simulink model "simulink_FCS_SDA"  (R2023a)
settings: Solver=VariableStepAuto  StartTime=0.0  StopTime=3*(1/freqHzSin)  FixedStep=Ts  RelTol=1e-3
InitFcn:
  | % try
  | %     Excel = actxGetRunningServer('Excel.Application');
  | %     Excel.ActiveWorkbook.Save;
  | %     Excel.ActiveWorkbook.Close(false);
  | % catch ExcelFechado
  | % end
StopFcn:
  | % t = table(out.seq, out.t_sim, 'VariableNames', ["Sequência de Vetores","Tempo de Simulação"]);
  | % writetable(t,'C:\Users\jpbru\OneDrive\Documentos\UFSC\COBEP 2023\sequencia_states.xlsx','Sheet','sim_CF_gw')
  | % winopen('C:\Users\jpbru\OneDrive\Documentos\UFSC\COBEP 2023\sequencia_states.xlsx')
  | %
  | % nome_arq = sprintf("gdq_caso-1_7.csv");
  | % writematrix([out.y_d out.y_q out.y_a out.y_b out.y_c out.ref_a out.ref_b out.ref_c],"C:\Users\jpbru\OneDrive\Documentos\MATLAB\CPBM\TrabFinal\Etapa 9 - Setembro2023 -\graficos\"+nome_arq)
  | 
  | sprintf("THD = %.3f", out.thd)
  | sprintf("MSE = %.3f", out.mse)
  | sprintf("Csw = %.0f", out.csw)
  | sprintf("Tempo de Computo = %.3fms", out.tavg*1000)
undefined symbols (not defined in the file or in its folder): A, B, Csim, dimA, dimB, DiscIntNeverNeededParam, freqHzSin, Lfilter, Lsim, N, N1, N2, Nu, Rsim, states, Ts, Vdc, Vdc_sim, Vnoise, Vref_pico, x_enb
libraries: dspstat3 x9, spsSeriesRLCBranchLib x9, spsVoltageMeasurementLib x7, spsIdealSwitchLib x6, spsTHDLib x4, simulink x2, spsabctoAlphaBetaZeroLib x2, spsAlphaBetaZerotoabcLib x1, spsControlledVoltageSourceLib x1, spspowerguiLib x1
settings Model: Creator=jpbru  LastModifiedBy=jpbru
settings SolverCC: AlgebraicLoopSolver=TrustRegion
settings DebuggingCC: UnconnectedInputMsg=warning  UnconnectedOutputMsg=warning  UnconnectedLineMsg=warning
settings ModelReferenceCC: EnableRefExpFcnMdlSchedulingChecks=on

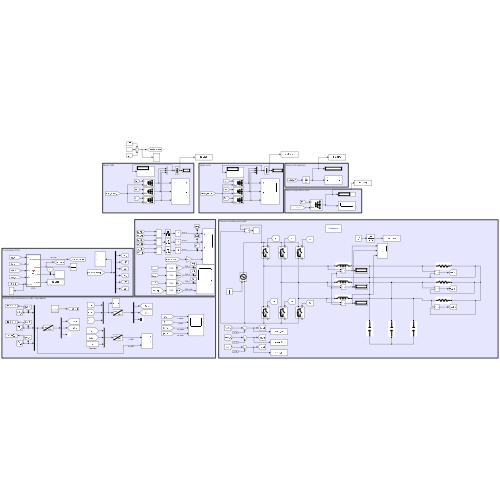
[thumbnail: Simulink's stored preview of the top-level diagram]
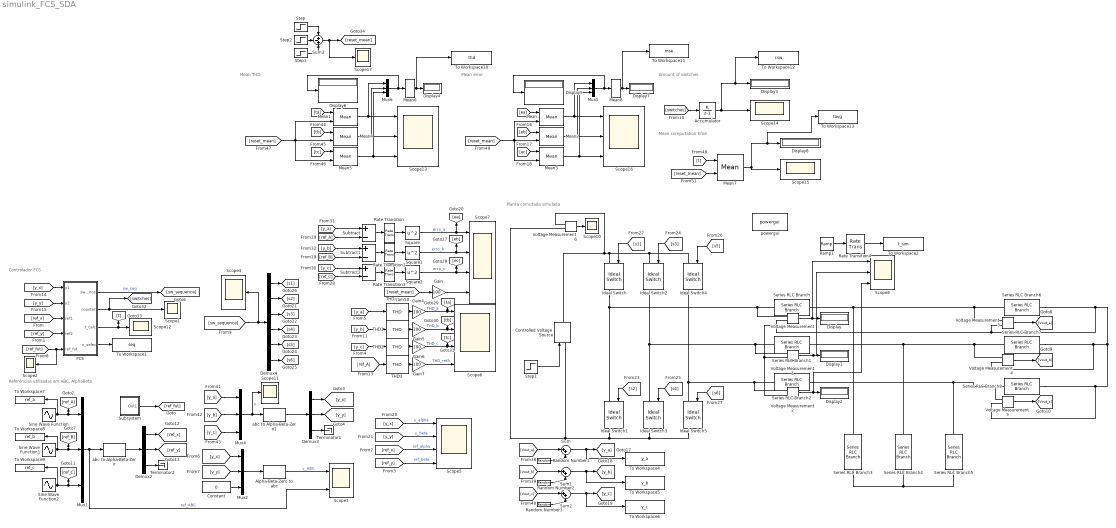
== system simulink_FCS_SDA ==
  note: Planta comutada simulada
  note: Referências utilizadas em ABC, AlphaBeta
  note: Controlador FCS
  note: Mean computation time
  note: Mean error
  note: Amount of switches
  note: Mean THD
  Accumulator : DiscreteIntegrator  IntegratorMethod=Accumulation: Forward Euler  SampleTime=-1  ICPrevOutput=DiscIntNeverNeededParam  ICPrevScaledInput=DiscIntNeverNeededParam
  Alpha-Beta-Zero to abc : spsAlphaBetaZerotoabcLib/Alpha-Beta-Zero to abc
      settings: LibrarySourceBlock=|
      | sps_lib/Control/Alpha-Beta-Zero
      | to abc
  Constant : Constant  Value=0  VectorParams1D=off  SampleTime=-1
  Controlled Voltage Source : spsControlledVoltageSourceLib/Controlled Voltage Source  Initialize=on  Source_Type=DC  Amplitude=Vdc_sim  Phase=0  Frequency=0  Measurements=None
  Demux2 : Demux  Outputs=3
  Demux3 : Demux  Outputs=3
  Demux4 : Demux  Outputs=6
  Display{,1..8} (9 alike) : Display
      Display8 settings: Format=short_e
  FCS : MATLAB Function  TreatAsAtomicUnit=on  SystemSampleTime=Ts
  Gain{,4..7} (5 alike) : Gain  Gain=100
  Ideal Switch{,1..5} (6 alike) : spsIdealSwitchLib/Ideal Switch  Ron=0.001  Lon=0  IC=0  Rs=1e5  Cs=inf  Measurements=on
  Mean{,1..5,7} (7 alike) : dspstat3/Mean  run=on  reset_popup=Rising edge  directionMode=Each column  dimension=1  roiEnable=off  roiType=Rectangles  roiPortion=Entire ROI  roiOutput=Individual statistics for each ROI  roiFlag=off  roundingMode=Floor  overflowMode=off  outputDataTypeStr=Inherit: Same as accumulator  outputMin=[]  outputMax=[]  outputLastDataTypeStr=Inherit: Same as accumulator
  Mean6 : dspstat3/Mean  run=off  reset_popup=Rising edge  directionMode=Entire input  dimension=1  roiEnable=off  roiType=Rectangles  roiPortion=Entire ROI  roiOutput=Individual statistics for each ROI  roiFlag=off  roundingMode=Floor  overflowMode=off  outputDataTypeStr=Inherit: Same as accumulator  outputMin=[]  outputMax=[]  outputLastDataTypeStr=Inherit: Same as accumulator
  Mean8 : dspstat3/Mean  run=off  reset_popup=Rising edge  directionMode=Entire input  dimension=1  roiEnable=off  roiType=Rectangles  roiPortion=Entire ROI  roiOutput=Individual statistics for each ROI  roiFlag=off  roundingMode=Floor  overflowMode=off  outputDataTypeStr=Inherit: Same as accumulator  outputMin=[]  outputMax=[]  outputLastDataTypeStr=Inherit: Same as accumulator
  Mux{1..2,4..6} (5 alike) : Mux  Inputs=3
  Ramp1 : simulink/Sources/Ramp  slope=1  start=0  InitialOutput=0
  Random Number1 : RandomNumber  Variance=Vnoise  SampleTime=Ts
  Random Number2 : RandomNumber  Variance=Vnoise  SampleTime=Ts
  Random Number3 : RandomNumber  Variance=Vnoise  SampleTime=Ts
  Rate Transition{,2..4} (4 alike) : RateTransition  OutPortSampleTime=Ts
  Scope{1..2,4,10..12,14..15,17} (9 alike) : Scope
  Scope13 : Scope  NumInputPorts=3
  Scope16 : Scope  NumInputPorts=3
  Scope3 : Scope  NumInputPorts=2
  Scope5 : Scope  NumInputPorts=4
  Scope6 : Scope  NumInputPorts=4
  Scope7 : Scope  NumInputPorts=4
  Scope8 : Scope  NumInputPorts=3
  Series RLC Branch : spsSeriesRLCBranchLib/Series RLC Branch  LConnTagsString=__new0  RConnTagsString=__new0  BranchType=L  Resistance=1  Inductance=Lsim  SetiL0=off  InitialCurrent=0  Capacitance=1e-6  Setx0=off  InitialVoltage=0  Measurements=None
  Series RLC Branch1 : spsSeriesRLCBranchLib/Series RLC Branch  LConnTagsString=__new0  RConnTagsString=__new0  BranchType=L  Resistance=1  Inductance=Lsim  SetiL0=off  InitialCurrent=0  Capacitance=1e-6  Setx0=off  InitialVoltage=0  Measurements=None
  Series RLC Branch2 : spsSeriesRLCBranchLib/Series RLC Branch  LConnTagsString=__new0  RConnTagsString=__new0  BranchType=L  Resistance=1  Inductance=Lsim  SetiL0=off  InitialCurrent=0  Capacitance=1e-6  Setx0=off  InitialVoltage=0  Measurements=None
  Series RLC Branch3 : spsSeriesRLCBranchLib/Series RLC Branch  LConnTagsString=__new0  RConnTagsString=__new0  BranchType=C  Resistance=1  Inductance=1e-3  SetiL0=off  InitialCurrent=0  Capacitance=Csim  Setx0=off  InitialVoltage=0  Measurements=None
  Series RLC Branch4 : spsSeriesRLCBranchLib/Series RLC Branch  LConnTagsString=__new0  RConnTagsString=__new0  BranchType=C  Resistance=1  Inductance=1e-3  SetiL0=off  InitialCurrent=0  Capacitance=Csim  Setx0=off  InitialVoltage=0  Measurements=None
  Series RLC Branch5 : spsSeriesRLCBranchLib/Series RLC Branch  LConnTagsString=__new0  RConnTagsString=__new0  BranchType=C  Resistance=1  Inductance=1e-3  SetiL0=off  InitialCurrent=0  Capacitance=Csim  Setx0=off  InitialVoltage=0  Measurements=None
  Series RLC Branch6 : spsSeriesRLCBranchLib/Series RLC Branch  LConnTagsString=__new0  RConnTagsString=__new0  BranchType=R  Resistance=Rsim  Inductance=Lfilter  SetiL0=off  InitialCurrent=0  Capacitance=1e-6  Setx0=off  InitialVoltage=0  Measurements=None
  Series RLC Branch7 : spsSeriesRLCBranchLib/Series RLC Branch  LConnTagsString=__new0  RConnTagsString=__new0  BranchType=R  Resistance=Rsim  Inductance=Lfilter  SetiL0=off  InitialCurrent=0  Capacitance=1e-6  Setx0=off  InitialVoltage=0  Measurements=None
  Series RLC Branch8 : spsSeriesRLCBranchLib/Series RLC Branch  LConnTagsString=__new0  RConnTagsString=__new0  BranchType=R  Resistance=Rsim  Inductance=Lfilter  SetiL0=off  InitialCurrent=0  Capacitance=1e-6  Setx0=off  InitialVoltage=0  Measurements=None
  Sine Wave Function : Sin  Amplitude=Vref_pico  Frequency=2*pi*50  SampleTime=Ts
  Sine Wave Function1 : Sin  Amplitude=Vref_pico  Frequency=2*pi*50  Phase=-2*pi/3  SampleTime=Ts
  Sine Wave Function2 : Sin  Amplitude=Vref_pico  Frequency=2*pi*50  Phase=2*pi/3  SampleTime=Ts
  Square : Math  Operator=square
  Square1 : Math  Operator=square
  Square2 : Math  Operator=square
  Step : Step  Time=(1/freqHzSin)  SampleTime=Ts
  Step1 : Step  Time=0.5  Before=Vdc_sim  After=Vdc_sim  SampleTime=Ts
  Step2 : Step  Time=(1/freqHzSin)+Ts  SampleTime=Ts
  Step3 : Step  Time=(1/freqHzSin)*2  SampleTime=Ts
  Subsystem : Subsystem
  Subtract : Sum  Inputs=+-
  Subtract1 : Sum  Inputs=+-
  Subtract2 : Sum  Inputs=+-
  Sum : Sum  Inputs=|++
  Sum1 : Sum  Inputs=|++
  Sum2 : Sum  Inputs=|++
  Sum3 : Sum  Inputs=+-+
  THD{,1..3} (4 alike) : spsTHDLib/THD  Freq=50  Ts=Ts
  Terminator1 : Terminator
  Terminator2 : Terminator
  To Workspace1 : ToWorkspace  VariableName=seq  SampleTime=Ts
      settings: Save2DSignal=2-D array (concatenate along first dimension)
  To Workspace10 : ToWorkspace  VariableName=thd  SampleTime=-1
      settings: MaxDataPoints=1
  To Workspace11 : ToWorkspace  VariableName=mse  SampleTime=-1
      settings: MaxDataPoints=1
  To Workspace12 : ToWorkspace  VariableName=csw  SampleTime=-1
      settings: MaxDataPoints=1
  To Workspace13 : ToWorkspace  VariableName=tavg  SampleTime=-1
      settings: MaxDataPoints=1
  To Workspace2 : ToWorkspace  VariableName=t_sim  SampleTime=Ts
      settings: Save2DSignal=2-D array (concatenate along first dimension)
  To Workspace4 : ToWorkspace  VariableName=y_a  SampleTime=Ts
      settings: Save2DSignal=2-D array (concatenate along first dimension)
  To Workspace5 : ToWorkspace  VariableName=y_b  SampleTime=Ts
      settings: Save2DSignal=2-D array (concatenate along first dimension)
  To Workspace6 : ToWorkspace  VariableName=y_c  SampleTime=Ts
      settings: Save2DSignal=2-D array (concatenate along first dimension)
  To Workspace7 : ToWorkspace  VariableName=ref_a  SampleTime=Ts
      settings: Save2DSignal=2-D array (concatenate along first dimension)
  To Workspace8 : ToWorkspace  VariableName=ref_b  SampleTime=Ts
      settings: Save2DSignal=2-D array (concatenate along first dimension)
  To Workspace9 : ToWorkspace  VariableName=ref_c  SampleTime=Ts
      settings: Save2DSignal=2-D array (concatenate along first dimension)
  Voltage Measurement{,1..6} (7 alike) : spsVoltageMeasurementLib/Voltage Measurement  PhasorSimulation=off  OutputType=Complex  PSBequivalent=0
  abc to Alpha-Beta-Zero : spsabctoAlphaBetaZeroLib/abc to Alpha-Beta-Zero
  abc to Alpha-Beta-Zero1 : spsabctoAlphaBetaZeroLib/abc to Alpha-Beta-Zero
  powergui : spspowerguiLib/powergui  Priority=1  SimulationMode=Continuous  SampleTime=Ts  frequency=60  Iterations=50  frequencyindice=0  Pbase=100e6  ErrMax=1e-4  UnitsV=kV  UnitsW=MW  buscounter=0  FunctionMessages=off  echomessages=off  EnableUseOfTLC=off  CurrentSourceSwitches=off  DisableSnubberDevices=off  DisableRonSwitches=off  DisableVfSwitches=off  DisplayEquations=off  AutomaticDiscreteSolvers=off  SolverType=Tustin/Backward Euler (TBE)  Interpol=off  ExternalGateDelay=off  methode=off  Ts=100  x0status=blocks  SPID=on  SwTol=0  HookPort=off  NonlinearTolerance=1e-4  nMaxIteration=100  ContinueOnMaxIteration=off  RestoreLinks=warning  ResistiveCurrentMeasurement=off  Frange=[0:2:500]  Ylog=off  Xlog=on  ShowGrid=off  save=off  variable=ZData  structure=0  ZoomFFT=off  StartTime=0.0  cycles=1  DisplayStyle=1  fundamental=60  FreqAxis=off  MaxFrequency=1000  frequencyindicesteady=1  RmsSteady=1  display=off
  wires:
  [ref_y] -> Scope5/4  "ref_beta"
  Sine Wave Function/1 -> Mux1/1, [ref_A], To Workspace7/1
  Sine Wave Function1/1 -> [ref_B], Mux1/2, To Workspace8/1
  Sine Wave Function2/1 -> [ref_C], Mux1/3, To Workspace9/1
  Mux1/1 -> Scope3/2, abc to Alpha-Beta-Zero/1  "ref_ABC"
  [y_x] -> Mux2/1
  [y_y] -> Mux2/2
  Constant/1 -> Mux2/3
  Alpha-Beta-Zero to abc/1 -> Scope3/1  "y_ABC"
  Voltage Measurement2/1 -> Scope8/3, Display2/1
  Voltage Measurement/1 -> Scope8/1, Display/1
  Voltage Measurement3/1 -> [Vout_a]
  Voltage Measurement4/1 -> [Vout_b]
  Voltage Measurement1/1 -> Scope8/2, Display1/1
  Voltage Measurement5/1 -> [Vout_c]
  [y_b] -> Mux4/2
  [y_a] -> Mux4/1
  [y_c] -> Mux4/3
  abc to Alpha-Beta-Zero1/1 -> Demux3/1
  Demux3/1 -> [y_x]
  Demux3/2 -> [y_y]
  [y_x] -> Scope5/1  "y_alpha"
  [y_y] -> Scope5/2  "y_beta"
  Demux3/3 -> Terminator1/1
  [s6] -> Ideal Switch5/1
  [s1] -> Ideal Switch/1
  [s2] -> Ideal Switch1/1
  [s3] -> Ideal Switch2/1
  [s5] -> Ideal Switch4/1
  [s4] -> Ideal Switch3/1
  Demux4/3 -> [s3]
  Demux4/1 -> [s1]
  Demux4/2 -> [s2]
  Demux4/5 -> [s5]
  Demux4/6 -> [s6]
  Demux4/4 -> [s4]
  [sw_sequence] -> Scope4/1, Demux4/1
  FCS/1(sw_sequence) -> [sw_sequence]  "sw_seq"
  [y_x] -> FCS/1(y1)
  [y_y] -> FCS/2(y2)
  [ref_x] -> FCS/3(ref1)
  [ref_y] -> FCS/4(ref2)
  FCS/2(counter) -> [switches], Scope1/1
  [ref_x] -> Scope5/3  "ref_alpha"
  Demux2/2 -> [ref_y]
  Demux2/1 -> [ref_x]
  Demux2/3 -> Terminator2/1
  abc to Alpha-Beta-Zero/1 -> Demux2/1
  Mux4/1 -> Scope11/1, abc to Alpha-Beta-Zero1/1  "y"
  Mux2/1 -> Alpha-Beta-Zero to abc/1
  Subsystem/1(Out1) -> [ref_fut]
  [ref_fut] -> Scope2/1, FCS/5(ref_fut)
  Voltage Measurement6/1 -> Scope10/1
  [Vout_b] -> Sum1/1
  Sum2/1 -> To Workspace6/1, [y_c]
  Sum/1 -> To Workspace4/1, [y_a]
  Random Number1/1 -> Sum/2
  Random Number2/1 -> Sum1/2
  Random Number3/1 -> Sum2/2
  Sum1/1 -> To Workspace5/1, [y_b]
  [Vout_a] -> Sum/1
  [Vout_c] -> Sum2/1
  FCS/3(t_calc) -> [t], Scope12/1
  [t] -> Mean7/1
  Mean7/1 -> To Workspace13/1, Display8/1, Scope15/1
  [ea] -> Mean/1
  [ec] -> Mean3/1
  Mux5/1 -> Mean8/1, Display5/1
  Mean/1 -> Mux5/1, Scope16/1
  Mean3/1 -> Mux5/3, Scope16/3
  Mean2/1 -> Mux5/2, Scope16/2
  [eb] -> Mean2/1
  THD/1 -> Gain4/1
  Square1/1 -> [eb], Scope7/2  "erro_b"
  [y_b] -> THD1/1
  [ref_B] -> Subtract1/2
  Gain5/1 -> [tb], Scope6/2  "THD_b"
  [y_c] -> Subtract2/1
  [y_b] -> Subtract1/1
  [ref_C] -> Subtract2/2
  [y_a] -> Subtract/1
  [ref_A] -> THD3/1
  THD1/1 -> Gain5/1
  Gain7/1 -> Scope6/4  "THD_refA"
  Subtract1/1 -> Rate Transition2/1
  THD2/1 -> Gain6/1
  Square2/1 -> [ec], Scope7/3  "erro_c"
  [ref_A] -> Subtract/2
  THD3/1 -> Gain7/1
  Gain6/1 -> [tc], Scope6/3  "THD_c"
  Subtract2/1 -> Rate Transition3/1
  [y_a] -> THD/1
  Subtract/1 -> Rate Transition/1
  Square/1 -> [ea], Scope7/1  "erro_a"
  [y_c] -> THD2/1
  Gain4/1 -> [ta], Scope6/1  "THD_a"
  Accumulator/1 -> To Workspace12/1, Display3/1, Scope14/1
  [switches] -> Accumulator/1
  [tc] -> Mean5/1
  [ta] -> Mean1/1
  Mean5/1 -> Mux6/3, Scope13/3
  Mean4/1 -> Mux6/2, Scope13/2
  [tb] -> Mean4/1
  Mux6/1 -> Display6/1, Mean6/1
  Mean1/1 -> Mux6/1, Scope13/1
  Rate Transition/1 -> Square/1
  Rate Transition2/1 -> Square1/1
  Rate Transition3/1 -> Square2/1
  [reset_mean] -> Mean1/2, Mean5/2, Mean4/2
  [reset_mean] -> Mean3/2, Mean2/2, Mean/2
  [reset_mean] -> Gain/1
  Gain/1 -> Scope7/4
  [reset_mean] -> Mean7/2
  Mean6/1 -> To Workspace10/1, Display4/1
  Mean8/1 -> To Workspace11/1, Display7/1
  Step1/1 -> Controlled Voltage Source/1
  FCS/4(x_selec) -> To Workspace1/1
  Ramp1/1 -> Rate Transition4/1
  Rate Transition4/1 -> To Workspace2/1
  Step/1 -> Sum3/1
  Step3/1 -> Sum3/3
  Step2/1 -> Sum3/2
  Sum3/1 -> Scope17/1, [reset_mean]
  connections:
  Ideal Switch3/LConn1 -- Ideal Switch2/RConn1 -- Voltage Measurement1/LConn1 -- Series RLC Branch1/LConn1
  Ideal Switch/RConn1 -- Ideal Switch1/LConn1 -- Voltage Measurement/LConn1 -- Series RLC Branch/LConn1
  Series RLC Branch6/RConn1 -- Voltage Measurement2/LConn2 -- Voltage Measurement1/LConn2 -- Voltage Measurement/LConn2 -- Voltage Measurement3/LConn2 -- Voltage Measurement4/LConn2 -- Series RLC Branch7/RConn1 -- Voltage Measurement5/LConn2 -- Series RLC Branch8/RConn1
  Ideal Switch5/LConn1 -- Ideal Switch4/RConn1 -- Voltage Measurement2/LConn1 -- Series RLC Branch2/LConn1
  Series RLC Branch3/RConn1 -- Series RLC Branch5/RConn1 -- Series RLC Branch4/RConn1
  Series RLC Branch/RConn1 -- Series RLC Branch3/LConn1 -- Series RLC Branch6/LConn1 -- Voltage Measurement3/LConn1
  Voltage Measurement5/LConn1 -- Series RLC Branch5/LConn1 -- Series RLC Branch2/RConn1 -- Series RLC Branch8/LConn1
  Voltage Measurement4/LConn1 -- Series RLC Branch4/LConn1 -- Series RLC Branch1/RConn1 -- Series RLC Branch7/LConn1
  Ideal Switch/LConn1 -- Controlled Voltage Source/RConn1 -- Voltage Measurement6/LConn1 -- Ideal Switch4/LConn1 -- Ideal Switch2/LConn1
  Ideal Switch1/RConn1 -- Controlled Voltage Source/LConn1 -- Voltage Measurement6/LConn2 -- Ideal Switch5/RConn1 -- Ideal Switch3/RConn1

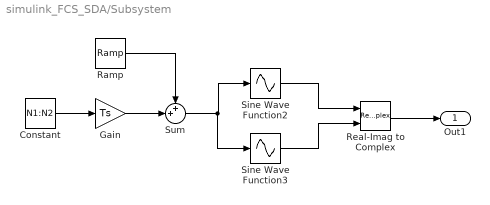
== system simulink_FCS_SDA/Subsystem ==
  Constant : Constant  Value=N1:N2
  Gain : Gain  Gain=Ts
  Ramp : simulink/Sources/Ramp  slope=1  start=0  InitialOutput=0
  Real-Imag to Complex : RealImagToComplex
  Sine Wave Function2 : Sin  TimeSource=Use external signal  Amplitude=Vref_pico  Frequency=2*pi*50  SampleTime=Ts
  Sine Wave Function3 : Sin  TimeSource=Use external signal  Amplitude=Vref_pico  Frequency=2*pi*50  Phase=-pi/2  SampleTime=Ts
  Sum : Sum  Inputs=++|
  Out1 : Outport
  wires:
  Sine Wave Function3/1 -> Real-Imag to Complex/2
  Sine Wave Function2/1 -> Real-Imag to Complex/1
  Sum/1 -> Sine Wave Function3/1, Sine Wave Function2/1
  Ramp/1 -> Sum/1
  Gain/1 -> Sum/2
  Real-Imag to Complex/1 -> Out1/1
  Constant/1 -> Gain/1

== matlab function simulink_FCS_SDA/FCS ==
  settings: updateMethod=DISCRETE  sampleTime=Ts
  data: y1 input; y2 input; ref1 input; ref2 input; ref_fut input size=N; dimA parameter; sw_sequence output; dimB parameter; states parameter; A parameter; Vdc parameter; counter output; Ts parameter; B parameter; t_calc output; N parameter; x_selec output; N1 parameter; Nu parameter; x_enb parameter
%function[variáveis que envia pra fora do bloco na simulação] = fcn(entradas(com conexões físicas) e parâmetros(que são pegos da workspace))
function [sw_sequence, counter, t_calc, x_selec] = fcn(y1, y2, ref1, ref2, ref_fut, dimA, dimB, states, A, Vdc, Ts, B, N, N1, Nu, x_enb) 
persistent t k pc pe1 pe2 pw1 pw2 y_ant u_ant a x_ant erro_intDQ u_ab %variáveis que mantém o valor entre os loops
if isempty(t) %caso t ainda não tenha valor definido
    t = 0; %o primeiro loop assume t=0
    k = 0; %variável que vai contar quantos loops são feitos para o cálculo de control
    
    %PARÂMETROS DE SINTONIZAÇÃO DO FCS-MPC
    pc = 0.35; %define o peso das comutações - quanto maior, menos comutações serão executadas durante o tempo de simulação 
    pe1 = 1; %define o peso do erro em D - quanto maior, menor deve ser o erro em D 
    pe2 = 1; %define o peso do erro em Q - quanto maior, menor deve ser o erro em Q 
    pw1 = 0; %define o peso do erro acumulado em D - quanto maior, menor deve ser o erro acumulado em D 
    pw2 = 0; %define o peso do erro acumulado em Q - quanto maior, menor deve ser o erro acumulado em Q

    a = exp(1j*(2*pi/3)); %define a variável que transforma os estados do inversor em uma variável complexa
    y_ant = complex(zeros(dimA-1,1)); %inicializa o vetor complexo com a memória das antigas saídas. (dimA-1) pois o primeiro termo é para a saída atual no polinômio. 
    u_ant = complex(zeros(dimB,1)); %inicializa o vetor complexo com a memória das antigas entradas.
    erro_intDQ = zeros(1,2); %inicializa o vetor do erro acumulado
    sw = complex((2/3)*(states(:,1)+a*states(:,2)+a^2*states(:,3))); %faz uma matriz com as variáveis complexas para cada combinação de estados
    u_ab = Vdc*sw; %multiplica a variável complexa dos estados das chaves com a tensão do barramento CC, resultando na matriz das tensões disponíveis em alphabeta 
    x_ant = 0; %inicializa a variável que armazena o último estado escolhido pelo último loop de controle
    for i = 1:size(x_enb,1) %bloco de repetição para definir o x_ant inicial
        if x_enb(i,1) ~= 0 %se for 0 passa pra próxima opção (evitar a linha dos nulos quando nulo = 0 por exemplo)
            x_ant = i; %x_ant assume o valor da linha que se encontra
            break; %encerra o loop for
        end
    end   
else %caso não seja o primeiro loop
    t = t + 1; %t vai incrementando em cada loop
    y_ant(end:-1:2) = y_ant(end-1:-1:1); %atualiza o vetor y_ant, passando os valores para uma linha abaixo da que estava  
end

% OBS: os comentários do tipo 1), 2), ... foram inspirados pelo artigo de
% Jin: "Model Predictive Voltage Control Based on Finite Control Set With 
% Computation Time Delay Compensation for PV Systems", e foram inseridos
% para facilitar a comparação entre o que deveria ser feito e o que estava
% sendo feito para a compensação do delay resultante do cálculo.

%-----------------------------------1) measurement of the load voltage and the actual error---------------------------------------
y = [y1 y2]'; %saída atual medida em k
vrefAB = [ref1 ref2]'; %referência atual que deveria estar a saída em k
wt = 2*pi*50*t*Ts; %posição angular em k
ab2dq = [sin(wt) -cos(wt); cos(wt) sin(wt)]; %Matriz que passa de alphabeta para DQ - 90 graus atrasada para o eixo d de DQ ser positivo
e_dq = (ab2dq*vrefAB - ab2dq*y)'; %erro atual em DQ
y_ant(1) = complex(y(1),y(2)); %armazena no vetor de saídas antigas

%-----------------------------------2) application of the switching state (calculated in the previous interval)-------------------
sw_sequence = zeros(6,1); %vetor que define o estado de cada uma das 6 chaves para aplicar nessa amostra
for aux = 1:3 %loop para definir o vetor
    sw_sequence(2*aux-1) = states(x_ant,aux); 
    sw_sequence(2*aux) = 1-states(x_ant,aux);
end

g_opt = inf; %inicializa variável que vai assumir o valor ótimo da função custo 
x_opt = 1; %inicializa variável que vai assumir o índice do vetor ótimo (o único aplicado) 

s_opt = []; %(APENAS PARA DEBUG) - inicializa variável que vai assumir a sequência ótima 
y_seq = complex(zeros(N,1)); %(APENAS PARA DEBUG) - inicializa variável que vai assumir a sequência de saídas preditas para cada sequência de entradas avaliada
x_seq = zeros(N,1); %inicializa variável auxiliar que vai assumir os índices da sequência de vetores avaliada
y_opt = y_seq; %(APENAS PARA DEBUG) - inicializa variável que vai assumir a sequência ótima de saídas preditas 

y_pred = complex(0); %inicializa variável auxiliar que vai assumir a saída predita em AB na forma complexa para cada opção avaliada em cada sequência
error = complex(0); %inicializa variável auxiliar que vai assumir o erro futuro entre a saída predita e a referência esperada naquela amostra de predição

t_inst = 0;  %inicializa variável que vai armazenar o tempo gasto pelo algoritmo para rodar o loop de controle
c_h1 = 0; %inicializa variável que vai armazenar quantas comutações serão aplicadas quando a opção ótima definida for implementada 

calc_vetor = true; %inicializa variável que define se o loop de cálculo da sequência ótima deve continuar ou não
pos_x = ones(N,1); %inicializa vetor que define a coluna em x_enb que cada amostra do horizonte está. Cada linha representa uma amostra. 

tic; %inicia a contagem de tempo do algoritmo de controle

%-----------------3) estimation of the value of the voltage at time tk+1, considering the applied switching state-----------------
y_est = complex(B*u_ant - A(2:end)*y_ant); %calcula a saída estimada em k+1 com base em sw_sequence que foi aplicado anteriormente nessa mesma amostra

%--------------4) prediction of the load voltages for the next sampling instant tk+2 for all possible switching states------------------
%-------------------------------------5) evaluation of the cost function for each prediction-------------------------------------------
erro_intDQ = erro_intDQ + e_dq; %calcula a integral do erro com base nos erros até k
while calc_vetor %inicia o loop que encontra o vetor ótimo a ser aplicado
    k = k+1;
    c = 0; %reseta/inicializa a variável que conta as comutações necessárias para implementar a sequência avaliada
    c1 = 0; %reseta/inicializa a variável que conta as comutações necessárias para implementar o primeiro vetor da sequência avaliada
    e1 = 0; %reseta/inicializa o erro quadrático no eixo D
    e2 = 0; %reseta/inicializa o erro quadrático no eixo Q
    w1 = 0; %reseta/inicializa o erro acumulado no eixo D
    w2 = 0; %reseta/inicializa o erro acumulado no eixo Q
    x_ant_aux = x_ant; %variável auxiliar para saber qual o estado que deve ser comparado para o cálculo de comutações e de onde parte o x_enb
    
     
    u_comp = u_ant; %vetor de entradas "antigas" (no ponto de vista da amostra predita) que será considerado para o cálculo da predição da saída
    y_comp = [y_est; y_ant(1:end-1)]; %vetor de saídas "antigas" (no ponto de vista da amostra predita) que será considerado para o cálculo da predição da saída
   
    for horizon = 1:N %inicializa uma variável horizon que representa a amostra que está sendo predita
        % if t==0 %(APENAS PARA DEBUG)
        %     sprintf("horizon = %.0f", horizon) %(APENAS PARA DEBUG)
        % end %(APENAS PARA DEBUG)
        % 
        % if t==0 %(APENAS PARA DEBUG)
        %     op_h = x_enb(1,pos_x(horizon)) %(APENAS PARA DEBUG)
        % else %(APENAS PARA DEBUG)
        op_h = x_enb(x_ant_aux,pos_x(horizon)); %armazena qual a linha de "states" definida nessa amostra
        % end %(APENAS PARA DEBUG)
        x_seq(horizon) = op_h; %insere a opção escolhida no vetor que armazena quais são as opções para cada amostra do horizonte

        if length(u_comp) > 1 %se u_comp não for escalar
            u_comp = [u_ab(op_h); u_comp(1:end-1)]; %atualizar o vetor com o novo u_ab considerado nessa amostra
        else %caso seja escalar
            u_comp = [u_ab(op_h)]; %apenas substituir 
        end
        y_pred = complex(B*u_comp - A(2:end)*y_comp); %calcula a saída predita na amostra

        y_seq(horizon) = y_pred; %(APENAS PARA DEBUG)

        wt = 2*pi*50*(t+horizon+N1-1)*Ts; %posição angular da amostra considerada
        ab2dq = [sin(wt) -cos(wt); cos(wt) sin(wt)]; %Matriz que passa de alphabeta para DQ - 90 graus atrasada para o d ser positivo
        
        error = ref_fut(horizon) - y_pred; %calcula o erro nessa amostra em alpha beta
        e_dq_fut = (ab2dq*[real(error);imag(error)])'; %transforma o erro para dq
        
        for col = 1:3 %faz um loop que passa entre as 3 colunas do states
            c = c + (abs(states(op_h,col) - states(x_ant_aux,col)))*2; %para cada coluna, se tiver alteração entre as linhas op_h e x_ant_aux de states, soma 2 para a contagem de c
        end
        
        if horizon == 1 %caso a amostra seja a primeira (aqui 1 não significa que é k+1, mas sim que é N1, assim como horizon = N significa que está em N2)
            c1 = c; %armazena as comutações necessárias para implementar o primeiro vetor da sequência avaliada
        end

        e1 = e1 + e_dq_fut(1)^2; %calcula o erro quadrático no eixo D
        e2 = e2 + e_dq_fut(2)^2; %calcula o erro quadrático no eixo Q
        w1 = w1 + e_dq_fut(1); %calcula o erro acumulado no eixo D
        w2 = w2 + e_dq_fut(2); %calcula o erro acumulado no eixo Q

        if horizon == N %se a amostra for a última considerada na predição (N2)
            w1 = erro_intDQ(1) + w1; %soma no erro acumulado predito o erro acumulado medido até a amostra k no eixo D
            w2 = erro_intDQ(2) + w2; %soma no erro acumulado predito o erro acumulado medido até a amostra k no eixo Q
            g = pe1*e1 + pe2*e2 + pw1*w1 + pw2*w2 + pc*c; %calcula a função custo
            % if t == 0 %(APENAS PARA DEBUG)
            %     x_seq %(APENAS PARA DEBUG)
            % end %(APENAS PARA DEBUG)
            if g < g_opt %se o valor da função custo for menor do que aquele que era o menor até então...
                g_opt = g; %... ele passa a ser o ótimo
                x_opt = x_seq(1); %a opção ótima que deve ser implementada passa a ser a primeira da sequência atual
                c_h1 = c1; %armazena a quantidade de comutações que a opção ótima vai requerir
                s_opt = pos_x; %(APENAS PARA DEBUG) %pega as posições em cada horizonte
                y_opt = y_seq; %(APENAS PARA DEBUG) %pega a sequência de saídas ótimas que a sequência ótima encontrou
            end
        else %se ainda não for a última amostra
            x_ant_aux = op_h; %atualiza a variável auxiliar que armazena qual foi o último estado no inversor
            y_comp = [y_pred; y_comp(1:end-1)]; %atualiza o vetor auxiliar utilizado no cálculo da saída predita, inserindo a saída que foi predita nesse loop dentro do vetor
        end
    end
    x_vet = [x_ant; x_seq]; %ao fim dos horizontes de predição, monta um vetor "x_vet" que possui as opções ótimas consideradas pela sequência ótima, em conjunto com o estado que o inversor definiu na amostra anterior
    for i = Nu:-1:1 %loop para atualizar pos_x e ir percorrendo todas as opções, entre N1 e N1+Nu
        pos_x(i) = pos_x(i) + 1; %começando por i=Nu, soma +1 na pos_x...
        if(x_enb(x_vet(i),pos_x(i)) == 0) %...mas se ela resultar em 0 dentro de x_enb...
            pos_x(i) = 1; %...reseta a pos_x e passa para Nu-1, assim por diante
        else 
            break; %caso não resulte em 0, o "for" é interrompido, pois a progressão é feita de um em um, partindo da amostra N1+Nu, indo até N1.
        end
        if i == 1 %se chegar aqui e entrar dentro do if significa que x_enb resultou em 0 para dado pos_x e i==1, então todas as opções já foram avaliadas (em dúvidas, plotar x_enb no script que ajuda pra entender) 
            calc_vetor = false; %muda a variável "calc_vetor" para "false", fazendo que quando finalizar o código, o loop while não vai rodar novamente
        end
    end
    pos_abs = x_ant; %enquanto pos_x é uma posição relativa (depende da linha anterior), a variável pos_abs é literalmente qual a opção escolhida em cada amostra do horizonte
    for i=1:Nu %loop para iteração de 1 para Nu 
        pos_abs = x_enb(pos_abs,pos_x(i)); %é uma variável pois deseja-se encontrar qual a posição absoluta em N1+Nu
    end
    if Nu<N %Caso o horizonte de controle seja menor que o de predição, precisa-se encontrar quais serão as opções consideradas para manter u_dq constante depois de Nu.
        wt = 2*pi*50*(t+1+Nu)*Ts; %acredito que tanto faz o tempo estar sincronizado, o que importa é ser o mesmo quando for voltar para ab, mas tentanto sincronizar: +1 por estar em k-1, +Nu para pegar a última considerada em k
        ab2dq = [sin(wt) -cos(wt); cos(wt) sin(wt)]; %matriz que passa de alphabeta para dq
        u_dq_Nu = (ab2dq*[real(u_ab(pos_abs));imag(u_ab(pos_abs))]); %encontra u_dq em Nu, com base na posição absoluta previamente encontrada
        for i = 1:N-Nu %para todas as amostras entre Nu e N
            wt = 2*pi*50*(t+1+Nu+i)*Ts; %atualiza a posição angular
            dq2ab = [sin(wt) cos(wt); -cos(wt) sin(wt)]; %matriz que transforma dq em alhpa beta
            u_ab_des = dq2ab*u_dq_Nu; %encontra qual seria o sinal em alpha beta desejado através do u_dq obtido em Nu, com a atualização de posição angular (preferi passar pra ab em vez de fazer em dq, pq desse jeito passo somenete a desejada para ab, e não todas as opções para dq)   
            conta_loop = 0; %conta qual opção está sendo considerada
            menor_erro_arred = inf; %variável semelhante com o q foi o g_opt anteriormente, mas focada em encontrar a opção que resulta no menor erro em dq com relação ao u_dq definido em Nu
            pos_abs_aux = 0; %inicializa uma variável que armazenará momentaneamente qual deverá ser a próxima posição absoluta
            for j = x_enb(pos_abs,:) %j assumirá todos os valores possíveis, partindo da linha da opção definida em Nu
                if j ~= 0 %caso não seja 0, ou seja, caso seja uma opção válida
                    conta_loop = conta_loop+1; %atualiza o contador de iterações, para saber qual coluna da linha pos_abs está sendo considerada
                    erro_arred_aux = (u_ab_des(1) - real(u_ab(j)))^2 + (u_ab_des(2) - imag(u_ab(j)))^2; %se menor_erro_arred é semelhante a g_opt, erro_arred_aux é como se fosse g, ou seja, uma função custo para definir qual opção aproxima mais ao que deveria ser um sinal constante em dq
                    if erro_arred_aux < menor_erro_arred %se a opçao trouxe o menor erro até o momento
                        menor_erro_arred = erro_arred_aux; %o menor erro a ser comparado passa a ser o dela
                        pos_abs_aux = j; %a posição absoluta auxiliar passa a ser a opção definida pelo for
                        pos_x(Nu+i) = conta_loop; %a posição relativa é correspondente ao contador de iterações
                    end
                else %se for 0, todas as opções da linha ja foram consideradas
                    break; %então pula pra próxima amostra, ou encerra o processo se for a última 
                end
            end
            pos_abs = pos_abs_aux; %utiliza pos_abs_aux para atualizar a posição absoluta considerada na próxima amostra
        end
    end
    % if t==0 %(APENAS PARA DEBUG)
    %     pos_x %(APENAS PARA DEBUG)
    % end %(APENAS PARA DEBUG)
end
% if t < 30 %(APENAS PARA DEBUG)
%     t %(APENAS PARA DEBUG)
%     y %(APENAS PARA DEBUG)
%     g_opt %(APENAS PARA DEBUG)
%     s_opt %(APENAS PARA DEBUG)
%     y_est %(APENAS PARA DEBUG)
%     y_opt %(APENAS PARA DEBUG)
% end %(APENAS PARA DEBUG)
t_inst = toc; %finaliza a contagem do tempo no código de controle FCS, e guarda na variável t_inst

% if t == 0 %(APENAS PARA DEBUG)
%     k %(APENAS PARA DEBUG)
% end %(APENAS PARA DEBUG)

u_ant(end:-1:2) = u_ant(end-1:-1:1); %atualiza o vetor de sinais de controle antigos
u_ant(1) = u_ab(x_opt); %o sinal mais recente no vetor passa a ser o que foi escolhido nesse loop de controle, mas ainda não é aplicado no sistema
%--------------------------------6) selection of the switching state that minimizes the cost function------------------------
x_ant = x_opt; %a opção anterior passa a ser a ótima desse loop de controle, para utilizar no próximo ciclo

counter = c_h1; %a variável que contará a quantidade de comutações associará a quantidade de comutações necessárias na primeira opção da sequência ótima
t_calc = t_inst; %o tempo de cáculo é passado para uma variável que envia para a simulação externa ao bloco
x_selec = x_opt - 1; %(APENAS PARA DEBUG) %para debug, subtrai-se 1 do valor de x_opt pois no livro base é de V0 a V7, não de V1 a V8, como feito aqui.
end
